simulink model "cordic_cosim"  (R2021a)
settings: Solver=VariableStepAuto  StartTime=0.0  StopTime=400  RelTol=1e-3
undefined symbols (not defined in the file or in its folder): A, N
libraries: hdlBasic x17, xbsIndex_r4 x1, JTAGRuntimeCosim_r4 x1
settings Model: Creator=hl116  LastModifiedBy=user

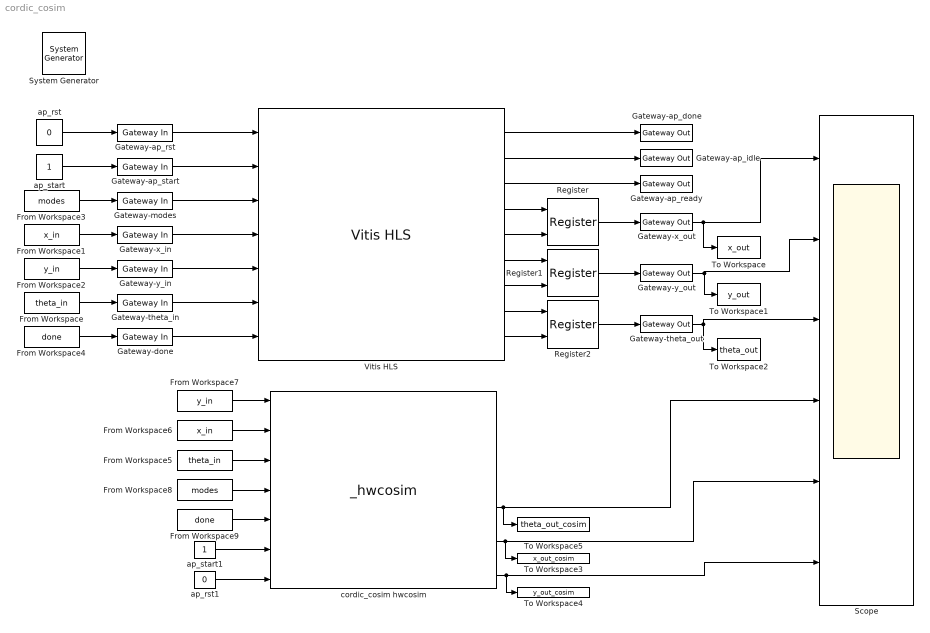
== system cordic_cosim ==
  " System Generator" : xbsIndex_r4/ System Generator  Tag=genX  xilinxfamily=zynq  part=xc7z020  speed=-1  package=clg484  synthesis_tool=Vivado  clock_wrapper=Clock Enables  directory=./netlist1  proj_type=Vivado  Synth_file=Vivado Synthesis Defaults  Impl_file=Vivado Implementation Defaults  testbench=off  simulink_period=1  sysclk_period=10  dcm_input_clock_period=10  incr_netlist=off  trim_vbits=Everywhere in SubSystem  dbl_ovrd=According to Block Masks  core_generation=According to Block Masks  run_coregen=off  deprecated_control=off  eval_field=0  block_type=sysgen
  From Workspace : FromWorkspace  VariableName=theta_in  Interpolate=off  OutputAfterFinalValue=Setting to zero
  From Workspace1 : FromWorkspace  VariableName=x_in  Interpolate=off  OutputAfterFinalValue=Setting to zero
  From Workspace2 : FromWorkspace  VariableName=y_in  Interpolate=off  OutputAfterFinalValue=Setting to zero
  From Workspace3 : FromWorkspace  VariableName=modes  Interpolate=off  OutputAfterFinalValue=Setting to zero
  From Workspace4 : FromWorkspace  VariableName=done  Interpolate=off  OutputAfterFinalValue=Setting to zero
  From Workspace5 : FromWorkspace  VariableName=theta_in  Interpolate=off  OutputAfterFinalValue=Setting to zero
  From Workspace6 : FromWorkspace  VariableName=x_in  Interpolate=off  OutputAfterFinalValue=Setting to zero
  From Workspace7 : FromWorkspace  VariableName=y_in  Interpolate=off  OutputAfterFinalValue=Setting to zero
  From Workspace8 : FromWorkspace  VariableName=modes  Interpolate=off  OutputAfterFinalValue=Setting to zero
  From Workspace9 : FromWorkspace  VariableName=done  Interpolate=off  OutputAfterFinalValue=Setting to zero
  Gateway-ap_done : hdlBasic/Gateway Out  inherit_from_input=off  hdl_port=on  rows=1  columns=1  UseAsDAC=off  DACChannel='1'  interface=None  automatic_assignment=on  address_offset=hex2dec('00')  intf_name=''  intf_description=''  timing_constraint=None  locs_specified=off  LOCs={}  io_standard={}  XmcBlockStatus=1  maskContainerNames=group4  block_type=gatewayout  block_config=sysgen:gateway_out_config  block_width_w=590  block_height_w=620  block_width=620  block_height=750
  Gateway-ap_idle : hdlBasic/Gateway Out  inherit_from_input=off  hdl_port=on  rows=1  columns=1  UseAsDAC=off  DACChannel='1'  interface=None  automatic_assignment=on  address_offset=hex2dec('00')  intf_name=''  intf_description=''  timing_constraint=None  locs_specified=off  LOCs={}  io_standard={}  XmcBlockStatus=1  maskContainerNames=group4  block_type=gatewayout  block_config=sysgen:gateway_out_config  block_width_w=590  block_height_w=620  block_width=620  block_height=750
  Gateway-ap_ready : hdlBasic/Gateway Out  inherit_from_input=off  hdl_port=on  rows=1  columns=1  UseAsDAC=off  DACChannel='1'  interface=None  automatic_assignment=on  address_offset=hex2dec('00')  intf_name=''  intf_description=''  timing_constraint=None  locs_specified=off  LOCs={}  io_standard={}  XmcBlockStatus=1  maskContainerNames=group4  block_type=gatewayout  block_config=sysgen:gateway_out_config  block_width_w=590  block_height_w=620  block_width=620  block_height=750
  Gateway-ap_rst : hdlBasic/Gateway In  gui_display_data_type=Boolean  arith_type=Boolean  n_bits=16  bin_pt=14  preci_type=Single  exp_width=8  frac_width=24  rows=1  columns=1  quantization="Round  (unbiased: +/- Inf)"  overflow=Saturate  period=1  UseAsADC=off  ADCChannel='1'  interface=None  automatic_assignment=on  address_offset=hex2dec('00')  intf_name=''  intf_description=''  default_value=0  timing_constraint=None  locs_specified=off  LOCs={}  io_standard={}  inherit_from_input=off  hdl_port=on  XmcBlockStatus=1  maskContainerNames=group4  block_type=gatewayin  block_config=sysgen:gateway_in_config  block_width_w=590  block_height_w=620  block_width=640  block_height=850
  Gateway-ap_start : hdlBasic/Gateway In  gui_display_data_type=Boolean  arith_type=Boolean  n_bits=16  bin_pt=14  preci_type=Single  exp_width=8  frac_width=24  rows=1  columns=1  quantization="Round  (unbiased: +/- Inf)"  overflow=Saturate  period=1  UseAsADC=off  ADCChannel='1'  interface=None  automatic_assignment=on  address_offset=hex2dec('00')  intf_name=''  intf_description=''  default_value=0  timing_constraint=None  locs_specified=off  LOCs={}  io_standard={}  inherit_from_input=off  hdl_port=on  XmcBlockStatus=1  maskContainerNames=group4  block_type=gatewayin  block_config=sysgen:gateway_in_config  block_width_w=590  block_height_w=620  block_width=640  block_height=850
  Gateway-done : hdlBasic/Gateway In  gui_display_data_type=Fixed-point  arith_type=Signed (2's comp)  n_bits=16  bin_pt=0  preci_type=Single  exp_width=8  frac_width=24  rows=1  columns=1  quantization="Round  (unbiased: +/- Inf)"  overflow=Saturate  period=1  UseAsADC=off  ADCChannel='1'  interface=None  automatic_assignment=on  address_offset=hex2dec('00')  intf_name=''  intf_description=''  default_value=0  timing_constraint=None  locs_specified=off  LOCs={}  io_standard={}  inherit_from_input=off  hdl_port=on  XmcBlockStatus=1  maskContainerNames=group4  block_type=gatewayin  block_config=sysgen:gateway_in_config  block_width_w=590  block_height_w=620  block_width=640  block_height=850
  Gateway-modes : hdlBasic/Gateway In  gui_display_data_type=Boolean  arith_type=Boolean  n_bits=16  bin_pt=12  preci_type=Single  exp_width=8  frac_width=24  rows=1  columns=1  quantization="Round  (unbiased: +/- Inf)"  overflow=Saturate  period=1  UseAsADC=off  ADCChannel='1'  interface=None  automatic_assignment=on  address_offset=hex2dec('00')  intf_name=''  intf_description=''  default_value=0  timing_constraint=None  locs_specified=off  LOCs={}  io_standard={}  inherit_from_input=off  hdl_port=on  XmcBlockStatus=1  maskContainerNames=group4  block_type=gatewayin  block_config=sysgen:gateway_in_config  block_width_w=590  block_height_w=620  block_width=640  block_height=850
  Gateway-theta_in : hdlBasic/Gateway In  gui_display_data_type=Fixed-point  arith_type=Signed (2's comp)  n_bits=16  bin_pt=12  preci_type=Single  exp_width=8  frac_width=24  rows=1  columns=1  quantization="Round  (unbiased: +/- Inf)"  overflow=Saturate  period=1  UseAsADC=off  ADCChannel='1'  interface=None  automatic_assignment=on  address_offset=hex2dec('00')  intf_name=''  intf_description=''  default_value=0  timing_constraint=None  locs_specified=off  LOCs={}  io_standard={}  inherit_from_input=off  hdl_port=on  XmcBlockStatus=1  maskContainerNames=group4  block_type=gatewayin  block_config=sysgen:gateway_in_config  block_width_w=590  block_height_w=620  block_width=640  block_height=850
  Gateway-theta_out : hdlBasic/Gateway Out  inherit_from_input=off  hdl_port=on  rows=1  columns=1  UseAsDAC=off  DACChannel='1'  interface=None  automatic_assignment=on  address_offset=hex2dec('00')  intf_name=''  intf_description=''  timing_constraint=None  locs_specified=off  LOCs={}  io_standard={}  XmcBlockStatus=1  maskContainerNames=group4  block_type=gatewayout  block_config=sysgen:gateway_out_config  block_width_w=590  block_height_w=620  block_width=620  block_height=750
  Gateway-x_in : hdlBasic/Gateway In  gui_display_data_type=Fixed-point  arith_type=Signed (2's comp)  n_bits=16  bin_pt=12  preci_type=Single  exp_width=8  frac_width=24  rows=1  columns=1  quantization="Round  (unbiased: +/- Inf)"  overflow=Saturate  period=1  UseAsADC=off  ADCChannel='1'  interface=None  automatic_assignment=on  address_offset=hex2dec('00')  intf_name=''  intf_description=''  default_value=0  timing_constraint=None  locs_specified=off  LOCs={}  io_standard={}  inherit_from_input=off  hdl_port=on  XmcBlockStatus=1  maskContainerNames=group4  block_type=gatewayin  block_config=sysgen:gateway_in_config  block_width_w=590  block_height_w=620  block_width=640  block_height=850
  Gateway-x_out : hdlBasic/Gateway Out  inherit_from_input=off  hdl_port=on  rows=1  columns=1  UseAsDAC=off  DACChannel='1'  interface=None  automatic_assignment=on  address_offset=hex2dec('00')  intf_name=''  intf_description=''  timing_constraint=None  locs_specified=off  LOCs={}  io_standard={}  XmcBlockStatus=1  maskContainerNames=group4  block_type=gatewayout  block_config=sysgen:gateway_out_config  block_width_w=590  block_height_w=620  block_width=620  block_height=750
  Gateway-y_in : hdlBasic/Gateway In  gui_display_data_type=Fixed-point  arith_type=Signed (2's comp)  n_bits=16  bin_pt=12  preci_type=Single  exp_width=8  frac_width=24  rows=1  columns=1  quantization="Round  (unbiased: +/- Inf)"  overflow=Saturate  period=1  UseAsADC=off  ADCChannel='1'  interface=None  automatic_assignment=on  address_offset=hex2dec('00')  intf_name=''  intf_description=''  default_value=0  timing_constraint=None  locs_specified=off  LOCs={}  io_standard={}  inherit_from_input=off  hdl_port=on  XmcBlockStatus=1  maskContainerNames=group4  block_type=gatewayin  block_config=sysgen:gateway_in_config  block_width_w=590  block_height_w=620  block_width=640  block_height=850
  Gateway-y_out : hdlBasic/Gateway Out  inherit_from_input=off  hdl_port=on  rows=1  columns=1  UseAsDAC=off  DACChannel='1'  interface=None  automatic_assignment=on  address_offset=hex2dec('00')  intf_name=''  intf_description=''  timing_constraint=None  locs_specified=off  LOCs={}  io_standard={}  XmcBlockStatus=1  maskContainerNames=group4  block_type=gatewayout  block_config=sysgen:gateway_out_config  block_width_w=590  block_height_w=620  block_width=620  block_height=750
  Register : hdlBasic/Register  init=0  rst=off  en=on  XmcBlockStatus=1  maskContainerNames=tabcontainer1  block_type=register  block_config=sysgen:Register_config
  Register1 : hdlBasic/Register  init=0  rst=off  en=on  XmcBlockStatus=1  maskContainerNames=tabcontainer1  block_type=register  block_config=sysgen:Register_config
  Register2 : hdlBasic/Register  init=0  rst=off  en=on  XmcBlockStatus=1  maskContainerNames=tabcontainer1  block_type=register  block_config=sysgen:Register_config
  Scope : Scope  NumInputPorts=6
  To Workspace : ToWorkspace  VariableName=x_out  SampleTime=-1
  To Workspace1 : ToWorkspace  VariableName=y_out  SampleTime=-1
  To Workspace2 : ToWorkspace  VariableName=theta_out  SampleTime=-1
  To Workspace3 : ToWorkspace  VariableName=x_out_cosim  SampleTime=-1
  To Workspace4 : ToWorkspace  VariableName=y_out_cosim  SampleTime=-1
  To Workspace5 : ToWorkspace  VariableName=theta_out_cosim  SampleTime=-1
  Vitis HLS : hdlBasic/Vitis HLS  anytable='C:\ELEC522\hl116\Project4\project4_v6\Vitis_HLS\project4_v6_hls\solution2-Optimized'  fast_sim=off  display_datatype=on  rate_propagation_method=Simulink system period  model_file_path=''  latency=1  block_type=vitis_hls
      settings: infoedit=This block allows including C,C++ and SystemC source files in System Generator for DSP designs.
  ap_rst : Constant  Value=0
  ap_rst1 : Constant  Value=0
  ap_start : Constant
  ap_start1 : Constant
  cordic_cosim hwcosim : JTAGRuntimeCosim_r4/_hwcosim  clkSrc=Single Stepped  hasCombinationalPath=on  bitfileName=C:\ELEC522\hl116\Project4\project4_v6\Model_Composer\netlist1\cordic_cosim.bit  skipConfig=off  dispPartInfo=off  useZynqReconfigScript=on  cable=Auto Detect  speed=N/A  cablePort=N/A  cableLocation=Local  shareCable=off  xmp=[]  software_settings=[]  design_xtable=|  binDir=[]  engineDll=JTAGCosimEngine.dll  cableWaitTime=10  bscanPos=-1  IRLengths=[]  useWaitBox=1  hasBufgmux=on  Scheme=Cosim  useCmdProc=1  hasProc=0  useImpact=0  printLogFile=0  userChain=2  XmcBlockStatus=0  maskContainerNames=tabcontainer1  block_type=jtagcosim  block_config=Sysgen:hwcosim_block_config
      | {
      |     'clkWrapper' => 'cordic_cosim',
      |     'burstMode' => false,
      |     'burstFifoDepth' => '1024',
      |     'shared_memories' => {},
      |     'clocksGcd' => 1,
      |     'device' => {
      |       'family' => 'zynq',
      |       'part' => 'xc7z020',
      |       'package' => 'clg484',
      |       'speed' => '-1',
      |     },
      |     'ports' => {
      |       'gateway_y_in' => {
      |         'direction' => 'in',
      |         'width' => 16,
      |         'name' => 'gateway_y_in',
      |         'period' => 1,
      |         'icon_text' => 'Gateway-y_in',
      |         'type' => 'Fix_16_12',
      |         'arithmetic_type' => 'xlSigned',
      |         'dat_file' => 'cordic_cosim_gateway_y_in.dat',
      |         'bin_pt' => 12,
      |         'addr_offset' => 0,
      |         'bd_port_index' => 0,
      |       },
      |       'gateway_x_in' => {
      |         'direction' => 'in',
      |         'width' => 16,
      |         'name' => 'gateway_x_in',
      |         'period' => 1,
      |         'icon_text' => 'Gateway-x_in',
      |         'type' => 'Fix_16_12',
      |         'arithmetic_type' => 'xlSigned',
      |         'dat_file' => 'cordic_cosim_gateway_x_in.dat',
      |         'bin_pt' => 12,
      |         'addr_offset' => 4,
      |         'bd_port_index' => 1,
      |       },
      |       'gateway_theta_in' => {
      |         'direction' => 'in',
      |         'width' => 16,
      |         'name' => 'gateway_theta_in',
      |         'period' => 1,
      |         'icon_text' => 'Gateway-theta_in',
      |         'type' => 'Fix_16_12',
      |         'arithmetic_type' => 'xlSigned',
      |         'dat_file' => 'cordic_cosim_gateway_theta_in.dat',
      |         'bin_pt' => 12,
      |         'addr_offset' => 8,
      |         'bd_port_index' => 2,
      |       },
      |       'gateway_modes' => {
      |         'direction' => 'in',
      |         'width' => 1,
      |         'name' => 'gateway_modes',
      |         'period' => 1,
      |         'icon_text' => 'Gateway-modes',
      |         'type' => 'Bool',
      |         'arithmetic_type' => 'xlUnsigned',
      |         'dat_file' => 'cordic_cosim_gateway_modes.dat',
      |         'bin_pt' => 0,
      |         'addr_offset' => 12,
      |         'bd_port_index' => 3,
      |       },
      |       'gateway_done' => {
      |         'direction' => 'in',
      |         'width' => 16,
      |         'name' => 'gateway_done',
      |         'period' => 1,
      |         'icon_text' => 'Gateway-done',
      |         'type' => 'Fix_16_0',
      |         'arithmetic_type' => 'xlSigned',
      |         'dat_file' => 'cordic_cosim_gateway_done.dat',
      |         'bin_pt' => 0,
      |         'addr_offset' => 16,
      |         'bd_port_index' => 4,
      |       },
      |       'gateway_ap_start' => {
      |         'direction' => 'in',
      |         'width' => 1,
      |         'name' => 'gateway_ap_start',
      |         'period' => 1,
      |         'icon_text' => 'Gateway-ap_start',
      |         'type' => 'Bool',
      |         'arithmetic_type' => 'xlUnsigned',
      |         'dat_file' => 'cordic_cosim_gateway_ap_start.dat',
      |         'bin_pt' => 0,
      |         'addr_offset' => 20,
      |         'bd_port_index' => 5,
      |       },
      |       'gateway_ap_rst' => {
      |         'direction' => 'in',
      |         'width' => 1,
      |         'name' => 'gateway_ap_rst',
      |         'period' => 1,
      |         'icon_text' => 'Gateway-ap_rst',
      |         'type' => 'Bool',
      |         'arithmetic_type' => 'xlUnsigned',
      |         'dat_file' => 'cordic_cosim_gateway_ap_rst.dat',
      |         'bin_pt' => 0,
      |         'addr_offset' => 24,
      |         'bd_port_index' => 6,
      |       },
      |       'gateway_ap_done' => {
      |         'direction' => 'out',
      |         'width' => 1,
      |         'name' => 'gateway_ap_done',
      |         'period' => 1,
      |         'icon_text' => 'Gateway-ap_done',
      |         'type' => 'Bool',
      |         'arithmetic_type' => 'xlUnsigned',
      |         'dat_file' => 'cordic_cosim_gateway_ap_done.dat',
      |         'bin_pt' => 0,
      |         'addr_offset' => 28,
      |         'bd_port_index' => 0,
      |       },
      |       'gateway_ap_idle' => {
      |         'direction' => 'out',
      |         'width' => 1,
      |         'name' => 'gateway_ap_idle',
      |         'period' => 1,
      |         'icon_text' => 'Gateway-ap_idle',
      |         'type' => 'Bool',
      |         'arithmetic_type' => 'xlUnsigned',
      |         'dat_file' => 'cordic_cosim_gateway_ap_idle.dat',
      |         'bin_pt' => 0,
      |         'addr_offset' => 32,
      |         'bd_port_index' => 1,
      |       },
      |       'gateway_ap_ready' => {
      |         'direction' => 'out',
      |         'width' => 1,
      |         'name' => 'gateway_ap_ready',
      |         'period' => 1,
      |         'icon_text' => 'Gateway-ap_ready',
      |         'type' => 'Bool',
      |         'arithmetic_type' => 'xlUnsigned',
      |         'dat_file' => 'cordic_cosim_gateway_ap_ready.dat',
      |         'bin_pt' => 0,
      |         'addr_offset' => 36,
      |         'bd_port_index' => 2,
      |       },
      |       'gateway_theta_out' => {
      |         'direction' => 'out',
      |         'width' => 16,
      |         'name' => 'gateway_theta_out',
      |         'period' => 1,
      |         'icon_text' => 'Gateway-theta_out',
      |         'type' => 'Fix_16_12',
      |         'arithmetic_type' => 'xlSigned',
      |         'dat_file' => 'cordic_cosim_gateway_theta_out.dat',
      |         'bin_pt' => 12,
      |         'addr_offset' => 40,
      |         'bd_port_index' => 3,
      |       },
      |       'gateway_x_out' => {
      |         'direction' => 'out',
      |         'width' => 16,
      |         'name' => 'gateway_x_out',
      |         'period' => 1,
      |         'icon_text' => 'Gateway-x_out',
      |         'type' => 'Fix_16_12',
      |         'arithmetic_type' => 'xlSigned',
      |         'dat_file' => 'cordic_cosim_gateway_x_out.dat',
      |         'bin_pt' => 12,
      |         'addr_offset' => 44,
      |         'bd_port_index' => 4,
      |       },
      |       'gateway_y_out' => {
      |         'direction' => 'out',
      |         'width' => 16,
      |         'name' => 'gateway_y_out',
      |         'period' => 1,
      |         'icon_text' => 'Gateway-y_out',
      |         'type' => 'Fix_16_12',
      |         'arithmetic_type' => 'xlSigned',
      |         'dat_file' => 'cordic_cosim_gateway_y_out.dat',
      |         'bin_pt' => 12,
      |         'addr_offset' => 48,
      |         'bd_port_index' => 5,
      |       },
      |     },
      |   }
  wires:
  Register/1 -> Gateway-x_out/1
  Gateway-ap_start/1 -> Vitis HLS/2
  Vitis HLS/5 -> Register/2
  Vitis HLS/4 -> Register/1
  Vitis HLS/1 -> Gateway-ap_done/1
  Vitis HLS/9 -> Register2/2
  Vitis HLS/3 -> Gateway-ap_ready/1
  ap_start/1 -> Gateway-ap_start/1
  Gateway-modes/1 -> Vitis HLS/3
  From Workspace1/1 -> Gateway-x_in/1
  Gateway-x_out/1 -> Scope/1, To Workspace/1
  From Workspace2/1 -> Gateway-y_in/1
  Gateway-done/1 -> Vitis HLS/7
  Vitis HLS/6 -> Register1/1
  Vitis HLS/2 -> Gateway-ap_idle/1
  Gateway-ap_rst/1 -> Vitis HLS/1
  ap_rst/1 -> Gateway-ap_rst/1
  Vitis HLS/7 -> Register1/2
  Gateway-theta_out/1 -> To Workspace2/1, Scope/3
  Gateway-y_out/1 -> To Workspace1/1, Scope/2
  From Workspace/1 -> Gateway-theta_in/1
  Register2/1 -> Gateway-theta_out/1
  Gateway-y_in/1 -> Vitis HLS/5
  Register1/1 -> Gateway-y_out/1
  Gateway-x_in/1 -> Vitis HLS/4
  Gateway-theta_in/1 -> Vitis HLS/6
  From Workspace3/1 -> Gateway-modes/1
  Vitis HLS/8 -> Register2/1
  From Workspace4/1 -> Gateway-done/1
  ap_rst1/1 -> cordic_cosim hwcosim/7
  ap_start1/1 -> cordic_cosim hwcosim/6
  From Workspace6/1 -> cordic_cosim hwcosim/2
  From Workspace7/1 -> cordic_cosim hwcosim/1
  From Workspace5/1 -> cordic_cosim hwcosim/3
  From Workspace8/1 -> cordic_cosim hwcosim/4
  From Workspace9/1 -> cordic_cosim hwcosim/5
  cordic_cosim hwcosim/6 -> Scope/6, To Workspace4/1
  cordic_cosim hwcosim/4 -> Scope/4, To Workspace5/1
  cordic_cosim hwcosim/5 -> To Workspace3/1, Scope/5
